simulink model "simulation"  (R2022a)
settings: Solver=VariableStepAuto  StartTime=0.0  StopTime=15  RelTol=1e-3
values from neighbouring files (symbols this model uses):
  p_goal = [0.15, 0.02, 0.05]    [main.m]
  p_inter = [0.1, 0.01, 0.04]    [main.m]
  p_start = [0.0, 0.0, 0.0]    [main.m]
  t_final = 10    [main.m]
libraries: slpidlib x3
settings Model: Creator=Dell  LastModifiedBy=Dell

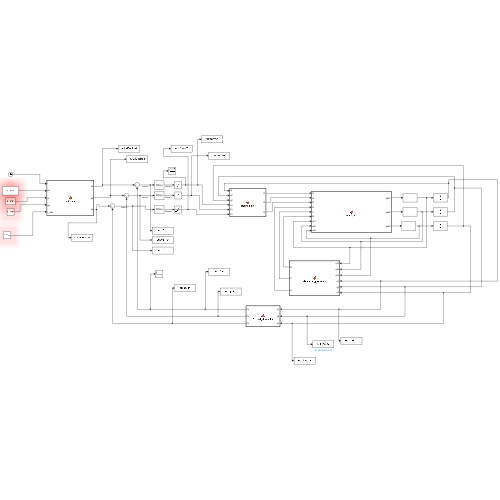
[thumbnail: Simulink's stored preview of the top-level diagram]
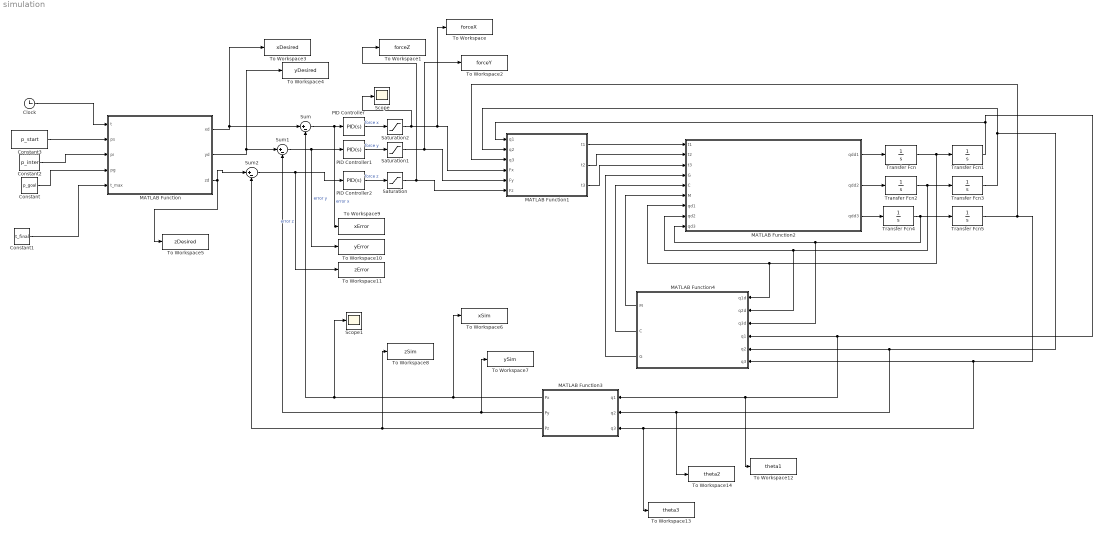
== system simulation ==
  Clock : Clock
  Constant : Constant  Value=p_goal
  Constant1 : Constant  Value=t_final
  Constant2 : Constant  Value=p_inter
  Constant3 : Constant  Value=p_start
  MATLAB Function : MATLAB Function  TreatAsAtomicUnit=on
  MATLAB Function1 : MATLAB Function  TreatAsAtomicUnit=on
  MATLAB Function2 : MATLAB Function  TreatAsAtomicUnit=on
  MATLAB Function3 : MATLAB Function  TreatAsAtomicUnit=on
  MATLAB Function4 : MATLAB Function  TreatAsAtomicUnit=on
  PID Controller : slpidlib/PID Controller  Controller=PID  Form=Parallel  TimeDomain=Continuous-time  UseExternalTs=off  SampleTime=-1  IntegratorMethod=Forward Euler  FilterMethod=Forward Euler  ControllerParametersSource=internal  P=60.326791  I=282.4185353  UseKiTs=off  D=3.1642482122  N=545.39702542169  UseFilter=on  TunerSelectOption=Transfer Function Based (PID Tuner App)  InitialConditionSource=internal  InitialConditionForIntegrator=0  InitialConditionForFilter=0  DifferentiatorICPrevScaledInput=0  ExternalReset=none  TrackingMode=off  Kt=1  LimitOutput=off  SatLimitsSource=internal  UpperSaturationLimit=1  LowerSaturationLimit=-1  LinearizeAsGain=on  AntiWindupMode=none  Kb=1  POutMin=[]  POutMax=[]  IOutMin=[]  IOutMax=[]  DOutMin=[]  DOutMax=[]  NOutMin=[]  NOutMax=[]  SumOutMin=[]  SumOutMax=[]  SaturationOutMin=[]  SaturationOutMax=[]  PParamMin=[]  PParamMax=[]  IParamMin=[]  IParamMax=[]  DParamMin=[]  DParamMax=[]  NParamMin=[]  NParamMax=[]  KbParamMin=[]  KbParamMax=[]  KtParamMin=[]  KtParamMax=[]  KbOutMin=[]  KbOutMax=[]  KtOutMin=[]  KtOutMax=[]  IntegratorOutMin=[]  IntegratorOutMax=[]  FilterOutMin=[]  FilterOutMax=[]  SumI1OutMin=[]  SumI1OutMax=[]  SumI2OutMin=[]  SumI2OutMax=[]  SumI3OutMin=[]  SumI3OutMax=[]  SumI4OutMin=[]  SumI4OutMax=[]  SumDOutMin=[]  SumDOutMax=[]  DifferentiatorOutMin=[]  DifferentiatorOutMax=[]  FilterDiffOutCoefMin=[]  FilterDiffOutCoefMax=[]  ReciprocalOutMin=[]  ReciprocalOutMax=[]  SumDenOutMin=[]  SumDenOutMax=[]  SumNumOutMin=[]  SumNumOutMax=[]  DivideOutMin=[]  DivideOutMax=[]  UdiffTsProdOutMin=[]  UdiffTsProdOutMax=[]  NTsProdOutMin=[]  NTsProdOutMax=[]  UintegralTsProdOutMin=[]  UintegralTsProdOutMax=[]  UngainTsProdOutMin=[]  UngainTsProdOutMax=[]  IntegratorContinuousStateAttributes=''  IntegratorStateMustResolveToSignalObject=off  IntegratorRTWStateStorageClass=Auto  FilterContinuousStateAttributes=''  FilterStateMustResolveToSignalObject=off  FilterRTWStateStorageClass=Auto  ParallelPVariant=InternalParameters  IdealPVariant=Disabled  IVariant=InternalParameters  DVariant=InternalParameters  IntegratorVariant=Continuous  SatVariant=Disabled  AWVariant=Passthrough  PCopyVariant=Disabled  TRVariant=Disabled  FdbkBlocksVariant=Forward  IdealPFdbkVariant=Disabled  SatFdbkVariant=Disabled  DerivativeFilterVariant=ContFilter  NVariant=InternalParameters  NCopyVariant=Disabled  FilterICVariant=InternalICsFilter  IntegratorICVariant=InternalICs  ExternalResetVariant=Disabled  TRSumVariant=Passthrough  SumFdbkVariant=Disabled  SumVariant=Sum_PID  TsampFilterVariant=InternalTs  TsampNgainVariant=Passthrough  TsampIntegralVariant=Passthrough  ExternalSaturationOutDataTypeStr=Inherit: Same as second input  aMode=0
  PID Controller1 : slpidlib/PID Controller  Controller=PID  Form=Parallel  TimeDomain=Continuous-time  UseExternalTs=off  SampleTime=-1  IntegratorMethod=Forward Euler  FilterMethod=Forward Euler  ControllerParametersSource=internal  P=97.4648679419947  I=456.27961827719  UseKiTs=off  D=5.11220683371593  N=545.397025421619  UseFilter=on  TunerSelectOption=Transfer Function Based (PID Tuner App)  InitialConditionSource=internal  InitialConditionForIntegrator=0  InitialConditionForFilter=0  DifferentiatorICPrevScaledInput=0  ExternalReset=none  TrackingMode=off  Kt=1  LimitOutput=off  SatLimitsSource=internal  UpperSaturationLimit=1  LowerSaturationLimit=-1  LinearizeAsGain=on  AntiWindupMode=none  Kb=1  POutMin=[]  POutMax=[]  IOutMin=[]  IOutMax=[]  DOutMin=[]  DOutMax=[]  NOutMin=[]  NOutMax=[]  SumOutMin=[]  SumOutMax=[]  SaturationOutMin=[]  SaturationOutMax=[]  PParamMin=[]  PParamMax=[]  IParamMin=[]  IParamMax=[]  DParamMin=[]  DParamMax=[]  NParamMin=[]  NParamMax=[]  KbParamMin=[]  KbParamMax=[]  KtParamMin=[]  KtParamMax=[]  KbOutMin=[]  KbOutMax=[]  KtOutMin=[]  KtOutMax=[]  IntegratorOutMin=[]  IntegratorOutMax=[]  FilterOutMin=[]  FilterOutMax=[]  SumI1OutMin=[]  SumI1OutMax=[]  SumI2OutMin=[]  SumI2OutMax=[]  SumI3OutMin=[]  SumI3OutMax=[]  SumI4OutMin=[]  SumI4OutMax=[]  SumDOutMin=[]  SumDOutMax=[]  DifferentiatorOutMin=[]  DifferentiatorOutMax=[]  FilterDiffOutCoefMin=[]  FilterDiffOutCoefMax=[]  ReciprocalOutMin=[]  ReciprocalOutMax=[]  SumDenOutMin=[]  SumDenOutMax=[]  SumNumOutMin=[]  SumNumOutMax=[]  DivideOutMin=[]  DivideOutMax=[]  UdiffTsProdOutMin=[]  UdiffTsProdOutMax=[]  NTsProdOutMin=[]  NTsProdOutMax=[]  UintegralTsProdOutMin=[]  UintegralTsProdOutMax=[]  UngainTsProdOutMin=[]  UngainTsProdOutMax=[]  IntegratorContinuousStateAttributes=''  IntegratorStateMustResolveToSignalObject=off  IntegratorRTWStateStorageClass=Auto  FilterContinuousStateAttributes=''  FilterStateMustResolveToSignalObject=off  FilterRTWStateStorageClass=Auto  ParallelPVariant=InternalParameters  IdealPVariant=Disabled  IVariant=InternalParameters  DVariant=InternalParameters  IntegratorVariant=Continuous  SatVariant=Disabled  AWVariant=Passthrough  PCopyVariant=Disabled  TRVariant=Disabled  FdbkBlocksVariant=Forward  IdealPFdbkVariant=Disabled  SatFdbkVariant=Disabled  DerivativeFilterVariant=ContFilter  NVariant=InternalParameters  NCopyVariant=Disabled  FilterICVariant=InternalICsFilter  IntegratorICVariant=InternalICs  ExternalResetVariant=Disabled  TRSumVariant=Passthrough  SumFdbkVariant=Disabled  SumVariant=Sum_PID  TsampFilterVariant=InternalTs  TsampNgainVariant=Passthrough  TsampIntegralVariant=Passthrough  ExternalSaturationOutDataTypeStr=Inherit: Same as second input  aMode=0
  PID Controller2 : slpidlib/PID Controller  Controller=PID  Form=Parallel  TimeDomain=Continuous-time  UseExternalTs=off  SampleTime=-1  IntegratorMethod=Forward Euler  FilterMethod=Forward Euler  ControllerParametersSource=internal  P=60.3267911825661  I=282.418535354203  UseKiTs=off  D=3.16424821221951  N=545.397025421619  UseFilter=on  TunerSelectOption=Transfer Function Based (PID Tuner App)  InitialConditionSource=internal  InitialConditionForIntegrator=0  InitialConditionForFilter=0  DifferentiatorICPrevScaledInput=0  ExternalReset=none  TrackingMode=off  Kt=1  LimitOutput=off  SatLimitsSource=internal  UpperSaturationLimit=1  LowerSaturationLimit=-1  LinearizeAsGain=on  AntiWindupMode=none  Kb=1  POutMin=[]  POutMax=[]  IOutMin=[]  IOutMax=[]  DOutMin=[]  DOutMax=[]  NOutMin=[]  NOutMax=[]  SumOutMin=[]  SumOutMax=[]  SaturationOutMin=[]  SaturationOutMax=[]  PParamMin=[]  PParamMax=[]  IParamMin=[]  IParamMax=[]  DParamMin=[]  DParamMax=[]  NParamMin=[]  NParamMax=[]  KbParamMin=[]  KbParamMax=[]  KtParamMin=[]  KtParamMax=[]  KbOutMin=[]  KbOutMax=[]  KtOutMin=[]  KtOutMax=[]  IntegratorOutMin=[]  IntegratorOutMax=[]  FilterOutMin=[]  FilterOutMax=[]  SumI1OutMin=[]  SumI1OutMax=[]  SumI2OutMin=[]  SumI2OutMax=[]  SumI3OutMin=[]  SumI3OutMax=[]  SumI4OutMin=[]  SumI4OutMax=[]  SumDOutMin=[]  SumDOutMax=[]  DifferentiatorOutMin=[]  DifferentiatorOutMax=[]  FilterDiffOutCoefMin=[]  FilterDiffOutCoefMax=[]  ReciprocalOutMin=[]  ReciprocalOutMax=[]  SumDenOutMin=[]  SumDenOutMax=[]  SumNumOutMin=[]  SumNumOutMax=[]  DivideOutMin=[]  DivideOutMax=[]  UdiffTsProdOutMin=[]  UdiffTsProdOutMax=[]  NTsProdOutMin=[]  NTsProdOutMax=[]  UintegralTsProdOutMin=[]  UintegralTsProdOutMax=[]  UngainTsProdOutMin=[]  UngainTsProdOutMax=[]  IntegratorContinuousStateAttributes=''  IntegratorStateMustResolveToSignalObject=off  IntegratorRTWStateStorageClass=Auto  FilterContinuousStateAttributes=''  FilterStateMustResolveToSignalObject=off  FilterRTWStateStorageClass=Auto  ParallelPVariant=InternalParameters  IdealPVariant=Disabled  IVariant=InternalParameters  DVariant=InternalParameters  IntegratorVariant=Continuous  SatVariant=Disabled  AWVariant=Passthrough  PCopyVariant=Disabled  TRVariant=Disabled  FdbkBlocksVariant=Forward  IdealPFdbkVariant=Disabled  SatFdbkVariant=Disabled  DerivativeFilterVariant=ContFilter  NVariant=InternalParameters  NCopyVariant=Disabled  FilterICVariant=InternalICsFilter  IntegratorICVariant=InternalICs  ExternalResetVariant=Disabled  TRSumVariant=Passthrough  SumFdbkVariant=Disabled  SumVariant=Sum_PID  TsampFilterVariant=InternalTs  TsampNgainVariant=Passthrough  TsampIntegralVariant=Passthrough  ExternalSaturationOutDataTypeStr=Inherit: Same as second input  aMode=0
  Saturation : Saturate  UpperLimit=1  LowerLimit=-1
  Saturation1 : Saturate  UpperLimit=1  LowerLimit=-1
  Saturation2 : Saturate  UpperLimit=1  LowerLimit=-1
  Scope : Scope
  Scope1 : Scope
  Sum : Sum  Inputs=|+-
  Sum1 : Sum  Inputs=|+-
  Sum2 : Sum  Inputs=|+-
  To Workspace : ToWorkspace  VariableName=forceX  SaveFormat=Timeseries  SampleTime=-1
  To Workspace1 : ToWorkspace  VariableName=forceZ  SaveFormat=Timeseries  SampleTime=-1
  To Workspace10 : ToWorkspace  VariableName=yError  SaveFormat=Timeseries  SampleTime=-1
  To Workspace11 : ToWorkspace  VariableName=zError  SaveFormat=Timeseries  SampleTime=-1
  To Workspace12 : ToWorkspace  VariableName=theta1  SaveFormat=Timeseries  SampleTime=-1
  To Workspace13 : ToWorkspace  VariableName=theta3  SaveFormat=Timeseries  SampleTime=-1
  To Workspace14 : ToWorkspace  VariableName=theta2  SaveFormat=Timeseries  SampleTime=-1
  To Workspace2 : ToWorkspace  VariableName=forceY  SaveFormat=Timeseries  SampleTime=-1
  To Workspace3 : ToWorkspace  VariableName=xDesired  SaveFormat=Timeseries  SampleTime=-1
  To Workspace4 : ToWorkspace  VariableName=yDesired  SaveFormat=Timeseries  SampleTime=-1
  To Workspace5 : ToWorkspace  VariableName=zDesired  SaveFormat=Timeseries  SampleTime=-1
  To Workspace6 : ToWorkspace  VariableName=xSim  SaveFormat=Timeseries  SampleTime=-1
  To Workspace7 : ToWorkspace  VariableName=ySim  SaveFormat=Timeseries  SampleTime=-1
  To Workspace8 : ToWorkspace  VariableName=zSim  SaveFormat=Timeseries  SampleTime=-1
  To Workspace9 : ToWorkspace  VariableName=xError  SaveFormat=Timeseries  SampleTime=-1
  Transfer Fcn{,1..5} (6 alike) : TransferFcn  Denominator=[1 0]
  wires:
  MATLAB Function/1(xd) -> To Workspace3/1, Sum/1
  MATLAB Function/2(yd) -> To Workspace4/1, Sum1/1
  MATLAB Function/3(zd) -> Sum2/1, To Workspace5/1
  Sum/1 -> To Workspace9/1, PID Controller/1  "error x"
  Sum2/1 -> To Workspace11/1, PID Controller2/1  "error z"
  Sum1/1 -> To Workspace10/1, PID Controller1/1  "error y"
  PID Controller/1 -> Saturation2/1  "force x"
  PID Controller1/1 -> Saturation1/1  "force y"
  PID Controller2/1 -> Saturation/1  "force z"
  MATLAB Function1/1(t1) -> MATLAB Function2/1(t1)
  MATLAB Function2/1(qdd1) -> Transfer Fcn/1
  Transfer Fcn/1 -> MATLAB Function4/1(q1d), MATLAB Function2/7(qd1), Transfer Fcn1/1
  MATLAB Function3/1(Px) -> To Workspace6/1, Scope1/1, Sum/2
  MATLAB Function3/2(Py) -> To Workspace7/1, Sum1/2
  MATLAB Function3/3(Pz) -> To Workspace8/1, Sum2/2
  MATLAB Function4/1(M) -> MATLAB Function2/6(M)
  MATLAB Function4/2(C) -> MATLAB Function2/5(C)
  MATLAB Function4/3(G) -> MATLAB Function2/4(G)
  MATLAB Function1/2(t2) -> MATLAB Function2/2(t2)
  MATLAB Function1/3(t3) -> MATLAB Function2/3(t3)
  MATLAB Function2/2(qdd2) -> Transfer Fcn2/1
  Transfer Fcn2/1 -> MATLAB Function4/2(q2d), MATLAB Function2/8(qd2), Transfer Fcn3/1
  MATLAB Function2/3(qdd3) -> Transfer Fcn4/1
  Transfer Fcn4/1 -> MATLAB Function4/3(q3d), MATLAB Function2/9(qd3), Transfer Fcn5/1
  Transfer Fcn1/1 -> To Workspace12/1, MATLAB Function3/1(q1), MATLAB Function4/4(q1), MATLAB Function1/1(q1)
  Transfer Fcn3/1 -> To Workspace14/1, MATLAB Function3/2(q2), MATLAB Function4/5(q2), MATLAB Function1/2(q2)
  Transfer Fcn5/1 -> To Workspace13/1, MATLAB Function3/3(q3), MATLAB Function4/6(q3), MATLAB Function1/3(q3)
  Clock/1 -> MATLAB Function/1(t)
  Saturation/1 -> To Workspace1/1, MATLAB Function1/6(Fz)
  Saturation2/1 -> Scope/1, To Workspace/1, MATLAB Function1/4(Fx)
  Saturation1/1 -> To Workspace2/1, MATLAB Function1/5(Fy)
  Constant1/1 -> MATLAB Function/5(t_max)
  Constant3/1 -> MATLAB Function/2(ps)
  Constant2/1 -> MATLAB Function/3(pi)
  Constant/1 -> MATLAB Function/4(pg)

== matlab function simulation/MATLAB Function1 ==
  data: q1 input; q2 input; q3 input; t1 output; Fx input; Fy input; Fz input; t2 output; t3 output
function [t1,t2,t3] = jacobian_pro(q1,q2,q3,Fx,Fy,Fz)
%#codegen

L1 = 0.215;%new
L2 = 0.170;

% Partial derivatives of Px, Py, and Pz with respect to q1, q2, and q3
dPx_dq1 = cos(q1)*(L1*cos(q2) + L2*sin(q3));
dPx_dq2 = -sin(q1)*sin(q2)*L1;
dPx_dq3 = sin(q1)*(L2*cos(q3));

dPy_dq1 = 0;
dPy_dq2 = L1*cos(q2);
dPy_dq3 = L2*sin(q3);

dPz_dq1 = -sin(q1)*(L1*cos(q2) + L2*sin(q3));
dPz_dq2 = -L1*sin(q2)*cos(q1);
dPz_dq3 = L2*cos(q3)*cos(q1);

% Jacobian matrix
J = [dPx_dq1, dPx_dq2, dPx_dq3;
     dPy_dq1, dPy_dq2, dPy_dq3;
     dPz_dq1, dPz_dq2, dPz_dq3];

torque = transpose(J) * [Fx; Fy; Fz];
t1 = torque(1);
t2 = torque(2);
t3 = torque(3);

== matlab function simulation/MATLAB Function ==
  data: t input; ps input; pi input; pg input; xd output; yd output; zd output; t_max input
function [xd, yd, zd] = path_pro(t,ps, pi, pg,t_max)
    % Calculate the number of points for each segment
    num_points_segment1 = 2000;
    num_points_segment2 = 2000;

    % Initialize arrays to store the coordinates
    xda = zeros(1, num_points_segment1 + num_points_segment2);
    yda = zeros(1, num_points_segment1 + num_points_segment2);
    zda = zeros(1, num_points_segment1 + num_points_segment2);

    % Generate the first segment from ps to pi
    xda(1:num_points_segment1) = linspace(ps(1), pi(1), num_points_segment1);
    yda(1:num_points_segment1) = linspace(ps(2), pi(2), num_points_segment1);
    zda(1:num_points_segment1) = linspace(ps(3), pi(3), num_points_segment1);

    % Generate the second segment from pi to pg
    xda(num_points_segment1+1:end) = linspace(pi(1), pg(1), num_points_segment2);
    yda(num_points_segment1+1:end) = linspace(pi(2), pg(2), num_points_segment2);
    zda(num_points_segment1+1:end) = linspace(pi(3), pg(3), num_points_segment2);
    
    if t < t_max
    %currentIndex = round(t * ((num_points_segment1 + num_points_segment2) - 1) / (t_max) + 1);
    currentIndex = round(t / (t_max) * (num_points_segment1 + num_points_segment2)) + 1;
    if currentIndex > (num_points_segment1 + num_points_segment2)
        currentIndex = num_points_segment1 + num_points_segment2;
    end

    xd = xda(currentIndex);
    yd = yda(currentIndex);
    zd = zda(currentIndex);

    else
        xd = xda(end);
        yd = yda(end);
        zd = zda(end);
    end


   
end

== matlab function simulation/MATLAB Function2 ==
  data: t1 input; t2 input; t3 input; G input; C input; M input; qd1 input; qd2 input; qd3 input; qdd1 output; qdd2 output; qdd3 output
function [qdd1,qdd2,qdd3] = robot_pro(t1,t2,t3,G,C,M,qd1,qd2,qd3)
torque = transpose([t1 t2 t3]);
qd = transpose([qd1*qd1 qd2*qd2 qd3*qd3]);

%torque = n x 1
% M => n x n  mass matrix
% V should be n x 1 but the given C is n x n


qdd = inv(M) * (torque - C * qd - G);

qdd1 = qdd(1);
qdd2 = qdd(2);
qdd3 = qdd(3);

== matlab function simulation/MATLAB Function3 ==
  data: q1 input; Px output; Py output; Pz output; q2 input; q3 input
function [Px,Py,Pz] = forward_kinematics(q1,q2,q3)
%#codegen
L1 = 0.215;
L2 = 0.170;
Px = sin(q1)*(L1*cos(q2) + L2 * sin(q3));
Py = L2 - L2 * cos(q3) + L1 * sin(q2);
Pz = -L1 + cos(q1)*(L1 * cos(q2) + L2 * sin(q3));

== matlab function simulation/MATLAB Function4 ==
  data: q1d input; q2d input; M output; C output; G output; q3d input; q1 input; q2 input; q3 input
function [M,C,G] = dynamical_properties(q1d,q2d,q3d,q1,q2,q3)

%q1 = q(1); q2 = q(2); q3 = q(3); 
%q1d = qd(1); q2d = qd(2); q3d = qd(3); 

%% phantom premium 1.5 parameters
ma = 0.0202;%new
mc = 0.0249;%new
mbe = 0.2359;%new
mdf = 0.1906;
l1 = 0.215;%new
l2 = 0.170;
l3 = 0.0325;
l5 = -36.8e-3;
l6 = 52.7e-3;
g = 9.81;

%% moment of inertia params
Iaxx = 0.4864e-4;
Iayy = 0.001843e-4;
Iazz = 0.4864e-4;
Icxx = 0.959e-4;
Icyy = 0.959e-4;
Iczz = 0.0051e-4;
Ibexx = 11.09e-4;
Ibeyy = 10.06e-4;
Ibezz = 0.591e-4;
Idfxx = 7.11e-4;
Idfyy = 0.629e-4;
Idfzz = 6.246e-4;
Ibaseyy = 11.87e-4;

%% mass matrix components
m11 = (0.125*(4*Iayy+4*Iazz+8*Ibaseyy+4*Ibeyy+4*Ibezz+4*Icyy+4*Iczz+4*Idfyy+4*Idfzz+4*l1*l1*ma+l2*l2*ma+l1*l1*mc+4*l3*l3*mc)...
    +0.125*(4*Ibeyy-4*Ibezz+4*Icyy-4*Iczz+l1*l1*(4*ma+mc))*cos(2*q2)...
    +0.125*(4*Iayy-4*Iazz+4*Idfyy-4*Idfzz-l2*l2*ma-4*l3*l3*mc)*cos(2*q3)+l1*(l2*ma+l3*mc)*cos(q2)*sin(q3));
m22 = 0.25*(4*(Ibexx+Icxx+l1*l1*ma)+l1*l1*mc);
m23 = -0.5*l1*(l2*ma+l3*mc)*sin(q2-q3);
m32 = m23;
m33 = 0.25*(4*Iaxx+4*Idfxx+l2*l2*ma+4*l3*l3*mc);

M = [m11 0 0;
    0 m22 m23;
    0 m32 m33];


%% coriolis matrix components
c11 = 0.125*(-2*sin(q2)*((4*Ibeyy-4*Ibezz+4*Icyy-4*Iczz+4*l1*l1*ma+l1*l1*mc)*cos(q2)+2*l1*(l2*ma+l3*mc)*sin(q3))*q2d...
    +2*cos(q3)*(2*l1*(l2*ma+l3*mc)*cos(q2)+(-4*Iayy+4*Iazz-4*Idfyy+4*Idfzz+l2*l2*ma+4*l3*l3*mc)*sin(q3))*q3d);
c12 = -0.125*((4*Ibeyy-4*Ibezz+4*Icyy-4*Iczz+l1*l1*(4*ma+mc))*sin(2*q2)+4*l1*(l2*ma+l3*mc)*sin(q2)*sin(q3))*q1d;
c13 = -0.125*(-4*l1*(l2*ma+l3*mc)*cos(q2)*cos(q3)-(-4*Iayy+4*Iazz-4*Idfyy+4*Idfzz+l2*l2*ma+4*l3*l3*mc)*sin(2*q3))*q1d;
c21 = -c12;
c22 = 0;
c23 = 0.5*l1*(l2*ma+l3*mc)*cos(q2-q3)*q3d;
c31 = -c13;
c32 = 0.5*l1*(l2*ma+l3*mc)*cos(q2-q3)*q2d;
c33 = 0;

C = [c11 c12 c13;
    c21 c22 c23;
    c31 c32 c33];

%% gravity vector components
tg1 = 0;
tg2 = g*(l1*(ma+0.5*mc)+l5*mbe)*cos(q2);
tg3 = g*(0.5*l2*ma+l3*mc-l6*mdf)*sin(q3);


G = [0;
    tg2;
    tg3];
